simulink model "Workshop_1"  (R2020b)
settings: Solver=VariableStepAuto  StartTime=0.0  StopTime=1  RelTol=1e-3
libraries: simulink x3
settings Model: Creator=linesLK  LastModifiedBy=linesLK

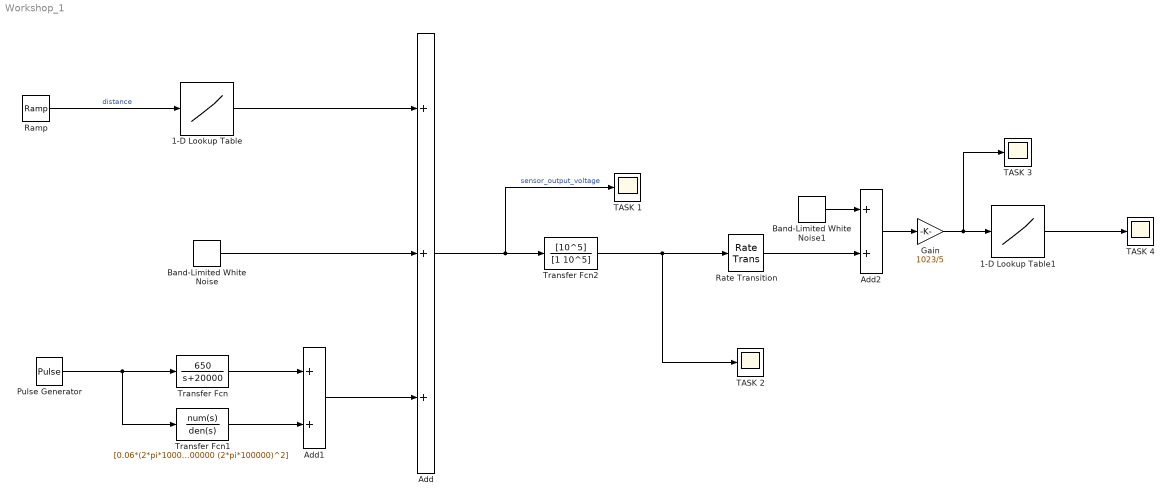
== system Workshop_1 ==
  1-D Lookup Table : Lookup_n-D  NumberOfTableDimensions=1  BreakpointsForDimension1=[0,10,15,20,30,40,50,60,70,80,90,100,110,120,130,140,150]/100  Table=[0,2.3,2.75,2.5,2,1.5,1.25,1.05,0.9,0.8,0.7,0.65,0.6,0.55,0.5,0.47,0.45]  InternalRulePriority=Speed  RndMeth=Simplest  InputSameDT=on
  1-D Lookup Table1 : Lookup_n-D  NumberOfTableDimensions=1  BreakpointsForDimension1=[0.45,0.47,0.5,0.55,0.6,0.65,0.7,0.8,0.9,1.05,1.25,1.5,2,2.5]*1023/5  Table=[150,140,130,120,110,100,90,80,70,60,50,40,30,20]*10  ExtrapMethod=Clip  InternalRulePriority=Speed  RndMeth=Simplest  InputSameDT=on
  Add : Sum  Inputs=+++
  Add1 : Sum
  Add2 : Sum
  Band-Limited White Noise : simulink/Sources/Band-Limited White Noise  Cov=[0.0000000001]  Ts=0.0001/125  seed=[23341]
  Band-Limited White Noise1 : simulink/Sources/Band-Limited White Noise  Cov=[0.000001]  Ts=0.1  seed=[23341]
  Gain : Gain  Gain=1023/5  OutDataTypeStr=uint16  SaturateOnIntegerOverflow=on
  Pulse Generator : DiscretePulseGenerator  PulseType=Time based  Amplitude=0.1  Period=0.001  PulseWidth=13
  Ramp : simulink/Sources/Ramp  slope=0.4  start=0  InitialOutput=0.2
  Rate Transition : RateTransition  OutPortSampleTime=0.1
  TASK {1..4} (4 alike) : Scope
  Transfer Fcn : TransferFcn  Numerator=[650]  Denominator=[1 20000]
  Transfer Fcn1 : TransferFcn  Numerator=[0.06*(2*pi*100000)^2]  Denominator=[1 4*0.3*pi*100000 (2*pi*100000)^2]
  Transfer Fcn2 : TransferFcn  Numerator=[10^5]  Denominator=[1 10^5]
  wires:
  1-D Lookup Table/1 -> Add/1
  Band-Limited White Noise/1 -> Add/2
  Pulse Generator/1 -> Transfer Fcn1/1, Transfer Fcn/1
  Transfer Fcn1/1 -> Add1/2
  Transfer Fcn/1 -> Add1/1
  Add1/1 -> Add/3
  Add/1 -> Transfer Fcn2/1, TASK 1/1  "sensor_output_voltage"
  Transfer Fcn2/1 -> Rate Transition/1, TASK 2/1
  Rate Transition/1 -> Add2/2
  Band-Limited White Noise1/1 -> Add2/1
  Add2/1 -> Gain/1
  Gain/1 -> TASK 3/1, 1-D Lookup Table1/1
  1-D Lookup Table1/1 -> TASK 4/1
  Ramp/1 -> 1-D Lookup Table/1  "distance"
